simulink model "loopback_exec"  (Simulink 3.00)
libraries: execlib x7

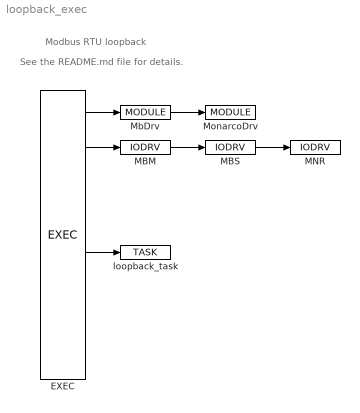
== system loopback_exec ==
  note: See the README.md file for details.
  note: Modbus RTU loopback
  EXEC : execlib/EXEC  target=Generic target device  tick=0.05  ntick0=10  ntick1=50  ntick2=100  ntick3=1200  pri0=5  pri1=9  pri2=13  pri3=18
  MBM : execlib/IODRV  module=MbDrv  classname=MbmDrv  cfgname=master_cfg.rio  factor=5  stack=10240  pri=3  timer=off
  MBS : execlib/IODRV  module=MbDrv  classname=MbsDrv  cfgname=slave_cfg.rio  factor=1  stack=10240  pri=3  timer=off
  MNR : execlib/IODRV  module=MonarcoDrv  classname=MonarcoHatDrv  cfgname=monarco.rio  factor=1  stack=10240  pri=3  timer=off
  MbDrv : execlib/MODULE
  MonarcoDrv : execlib/MODULE
  loopback_task : execlib/TASK  factor=1  start=0  stop=1  stack=10240  MDLOPEN=on
  wires:
  EXEC/1 -> MbDrv/1
  EXEC/2 -> MBM/1
  EXEC/5 -> loopback_task/1
  MBM/1 -> MBS/1
  MBS/1 -> MNR/1
  MbDrv/1 -> MonarcoDrv/1
